simulink model "brake_model"  (R2018b)
settings: Solver=FixedStepAuto  StartTime=0.0  StopTime=3  FixedStep=0.001  RelTol=1e-3
values from neighbouring files (symbols this model uses):
  a = 1.8    [formulacar_params.mat]    (also in longitudinal_coefficients.m; roadcar_params.mat = 1.1)
  A = 1.25    [formulacar_params.mat]    (also in longitudinal_coefficients.m; roadcar_params.mat = 1.8)
  a1 = -1e-5    (= -1e-05)    [longitudinal_coefficients.m]
  a2 = 1.25    [longitudinal_coefficients.m]
  b = 1.7    [formulacar_params.mat]    (also in longitudinal_coefficients.m; roadcar_params.mat)
  B = 4.1576    [longitudinal_coefficients.m]
  balance = 'understeer'    [bicycle_script.m]    (also in formulacar_params.mat; longitudinal_coefficients.m = 0.8; roadcar_params.mat)
  C = 1.7180    (= 1.718)    [longitudinal_coefficients.m]
  cd = 0.4    [longitudinal_coefficients.m]
  cz = 1    [formulacar_params.mat]    (also in longitudinal_coefficients.m; roadcar_params.mat = 0)
  g = 9.81    [formulacar_params.mat]    (also in longitudinal_coefficients.m; quarter_car_model_parameters.m; roadcar_params.mat)
  h = 0.2    [longitudinal_coefficients.m]
  Iwheel = 0.9    [longitudinal_coefficients.m]
  L = 3.5    [formulacar_params.mat]    (also in longitudinal_coefficients.m; roadcar_params.mat = 2.8)
  m = 850    [formulacar_params.mat]    (also in longitudinal_coefficients.m; roadcar_params.mat = 1650)
  r = 0.375    [longitudinal_coefficients.m]
  rbrake = 3800    [longitudinal_coefficients.m]
  rho = 1.225    [formulacar_params.mat]    (also in longitudinal_coefficients.m; roadcar_params.mat)
  V0 = 300    [longitudinal_coefficients.m]
settings Model: Creator=Cassio.Freitas  LastModifiedBy=Cassio.Freitas

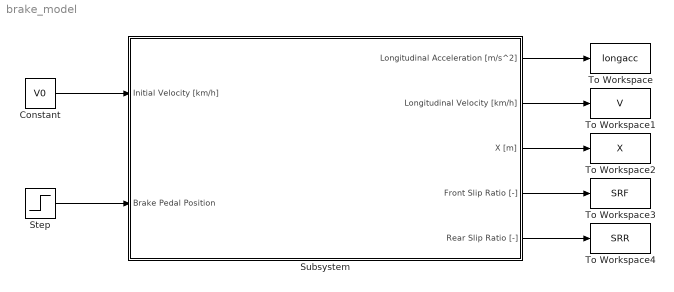
== system brake_model ==
  Constant : Constant  Value=V0
  Step : Step  SampleTime=0
  Subsystem : Subsystem
  To Workspace : ToWorkspace  VariableName=longacc  SaveFormat=Timeseries  SampleTime=-1
  To Workspace1 : ToWorkspace  VariableName=V  SaveFormat=Timeseries  SampleTime=-1
  To Workspace2 : ToWorkspace  VariableName=X  SaveFormat=Timeseries  SampleTime=-1
  To Workspace3 : ToWorkspace  VariableName=SRF  SaveFormat=Timeseries  SampleTime=-1
  To Workspace4 : ToWorkspace  VariableName=SRR  SaveFormat=Timeseries  SampleTime=-1
  wires:
  Constant/1 -> Subsystem/1(Initial Velocity [km/h])
  Step/1 -> Subsystem/2(Brake Pedal Position)
  Subsystem/1(Longitudinal Acceleration [m/s^2]) -> To Workspace/1
  Subsystem/2(Longitudinal Velocity [km/h]) -> To Workspace1/1
  Subsystem/3(X [m]) -> To Workspace2/1
  Subsystem/4(Front Slip Ratio [-]) -> To Workspace3/1
  Subsystem/5(Rear Slip Ratio [-]) -> To Workspace4/1

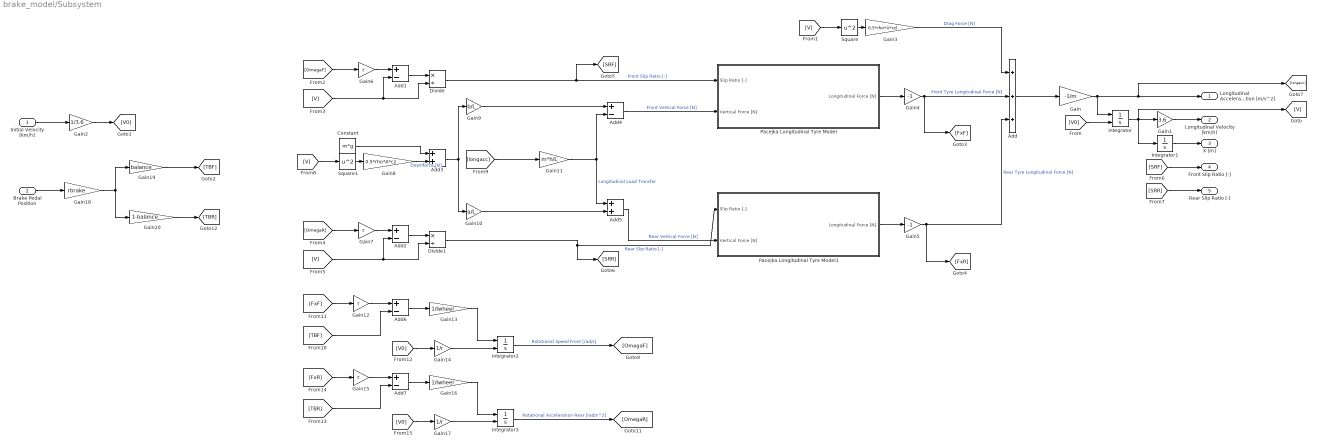
== system brake_model/Subsystem ==
  Initial Velocity [km/h] : Inport
  Brake Pedal Position : Inport  Port=2
  Add : Sum  Inputs=+++
  Add{1..2,4,6..7} (5 alike) : Sum  Inputs=+-
  Add3 : Sum
  Add5 : Sum
  Constant : Constant  Value=m*g
  Divide : Product  Inputs=*/
  Divide1 : Product  Inputs=*/
  Gain : Gain  Gain=-1/m
  Gain1 : Gain  Gain=3.6
  Gain10 : Gain  Gain=a/L
  Gain11 : Gain  Gain=m*h/L
  Gain{6..7,12,15} (4 alike) : Gain  Gain=r
  Gain13 : Gain  Gain=1/Iwheel
  Gain14 : Gain  Gain=1/r
  Gain16 : Gain  Gain=1/Iwheel
  Gain17 : Gain  Gain=1/r
  Gain18 : Gain  Gain=rbrake
  Gain19 : Gain  Gain=balance
  Gain2 : Gain  Gain=1/3.6
  Gain20 : Gain  Gain=1-balance
  Gain3 : Gain  Gain=0.5*rho*A*cd
  Gain4 : Gain  Gain=-1
  Gain5 : Gain  Gain=-1
  Gain8 : Gain  Gain=0.5*rho*A*cz
  Gain9 : Gain  Gain=b/L
  Integrator : Integrator  InitialConditionSource=external
  Integrator1 : Integrator
  Integrator2 : Integrator  InitialConditionSource=external
  Integrator3 : Integrator  InitialConditionSource=external
  Pacejka Longitudinal Tyre Model : Subsystem
  Pacejka Longitudinal Tyre Model1 : Subsystem
  Square : Math  Operator=square  SaturateOnIntegerOverflow=on
  Square1 : Math  Operator=square  SaturateOnIntegerOverflow=on
  Longitudinal Acceleration [m/s^2] : Outport
  Longitudinal Velocity [km/h] : Outport  Port=2
  X [m] : Outport  Port=3
  Front Slip Ratio [-] : Outport  Port=4
  Rear Slip Ratio [-] : Outport  Port=5
  wires:
  Gain/1 -> Integrator/1, [longacc], Longitudinal Acceleration [m/s^2]/1
  Add/1 -> Gain/1
  Integrator/1 -> [V], Integrator1/1, Gain1/1
  Gain1/1 -> Longitudinal Velocity [km/h]/1
  Integrator1/1 -> X [m]/1
  Initial Velocity [km/h]/1 -> Gain2/1
  Gain2/1 -> [V0]
  Brake Pedal Position/1 -> Gain18/1
  [V0] -> Integrator/2
  [V] -> Square/1
  Square/1 -> Gain3/1
  Gain3/1 -> Add/1  "Drag Force [N]"
  Pacejka Longitudinal Tyre Model/1(Longitudinal Force [N]) -> Gain4/1
  Gain4/1 -> [FxF], Add/2  "Front Tyre Longitudinal Force [N]"
  Pacejka Longitudinal Tyre Model1/1(Longitudinal Force [N]) -> Gain5/1
  Gain5/1 -> [FxR], Add/3  "Rear Tyre Longitudinal Force [N]"
  [OmegaF] -> Gain6/1
  Gain6/1 -> Add1/1
  [V] -> Divide/2, Add1/2
  Add1/1 -> Divide/1
  Divide/1 -> [SRF], Pacejka Longitudinal Tyre Model/1(Slip Ratio [-])  "Front Slip Ratio [-]"
  Add2/1 -> Divide1/1
  [V] -> Add2/2, Divide1/2
  Gain7/1 -> Add2/1
  [OmegaR] -> Gain7/1
  Divide1/1 -> Pacejka Longitudinal Tyre Model1/1(Slip Ratio [-]), [SRR]  "Rear Slip Ratio [-]"
  [SRF] -> Front Slip Ratio [-]/1
  [SRR] -> Rear Slip Ratio [-]/1
  Square1/1 -> Gain8/1
  [V] -> Square1/1
  Gain8/1 -> Add3/2  "Downforce [N]"
  Constant/1 -> Add3/1
  Add3/1 -> Gain10/1, Gain9/1
  Gain9/1 -> Add4/1
  Add4/1 -> Pacejka Longitudinal Tyre Model/2(Vertical Force [N])  "Front Vertical Force [N]"
  Gain10/1 -> Add5/2
  Gain11/1 -> Add5/1, Add4/2  "Longitudinal Load Transfer"
  Add5/1 -> Pacejka Longitudinal Tyre Model1/2(Vertical Force [N])  "Rear Vertical Force [N]"
  [FxF] -> Gain12/1
  Gain12/1 -> Add6/1
  [TBF] -> Add6/2
  Add6/1 -> Gain13/1
  Gain13/1 -> Integrator2/1
  Integrator2/1 -> [OmegaF]  "Rotational Speed Front [rad/s]"
  [V0] -> Gain14/1
  Gain14/1 -> Integrator2/2
  Gain17/1 -> Integrator3/2
  [V0] -> Gain17/1
  Integrator3/1 -> [OmegaR]  "Rotational Acceleration Rear [rad/s^2]"
  Gain16/1 -> Integrator3/1
  Add7/1 -> Gain16/1
  [TBR] -> Add7/2
  Gain15/1 -> Add7/1
  [FxR] -> Gain15/1
  Gain18/1 -> Gain20/1, Gain19/1
  Gain19/1 -> [TBF]
  Gain20/1 -> [TBR]
  [longacc] -> Gain11/1

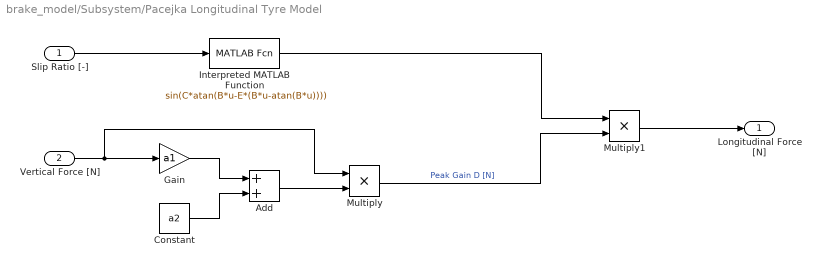
== system brake_model/Subsystem/Pacejka Longitudinal Tyre Model ==
  Slip Ratio [-] : Inport
  Vertical Force [N] : Inport  Port=2
  Add : Sum
  Constant : Constant  Value=a2
  Gain : Gain  Gain=a1
  Interpreted MATLAB Function : MATLABFcn  MATLABFcn=sin(C*atan(B*u-E*(B*u-atan(B*u))))
  Multiply : Product
  Multiply1 : Product
  Longitudinal Force [N] : Outport
  wires:
  Vertical Force [N]/1 -> Multiply/1, Gain/1
  Constant/1 -> Add/2
  Gain/1 -> Add/1
  Add/1 -> Multiply/2
  Multiply/1 -> Multiply1/2  "Peak Gain D [N]"
  Slip Ratio [-]/1 -> Interpreted MATLAB Function/1
  Interpreted MATLAB Function/1 -> Multiply1/1
  Multiply1/1 -> Longitudinal Force [N]/1

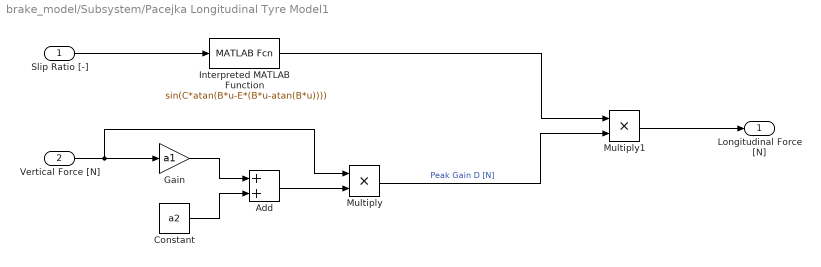
== system brake_model/Subsystem/Pacejka Longitudinal Tyre Model1 ==
  Slip Ratio [-] : Inport
  Vertical Force [N] : Inport  Port=2
  Add : Sum
  Constant : Constant  Value=a2
  Gain : Gain  Gain=a1
  Interpreted MATLAB Function : MATLABFcn  MATLABFcn=sin(C*atan(B*u-E*(B*u-atan(B*u))))
  Multiply : Product
  Multiply1 : Product
  Longitudinal Force [N] : Outport
  wires:
  Vertical Force [N]/1 -> Multiply/1, Gain/1
  Constant/1 -> Add/2
  Gain/1 -> Add/1
  Add/1 -> Multiply/2
  Multiply/1 -> Multiply1/2  "Peak Gain D [N]"
  Slip Ratio [-]/1 -> Interpreted MATLAB Function/1
  Interpreted MATLAB Function/1 -> Multiply1/1
  Multiply1/1 -> Longitudinal Force [N]/1
